simulink model "AC_Voltage_Controller"  (R2023b)
settings: Solver=VariableStepAuto  StartTime=0.0  StopTime=0.1  RelTol=1e-3
libraries: spsThyristorLib x6, spsCurrentMeasurementLib x4, spsRMSLib x4, spsVoltageMeasurementLib x4, spsSeriesRLCBranchLib x3, spsTHDLib x2, spsThreePhaseProgrammableVoltageSourceLib x1, sps_lib x1
settings Model: Creator=Anusha  LastModifiedBy=Anusha

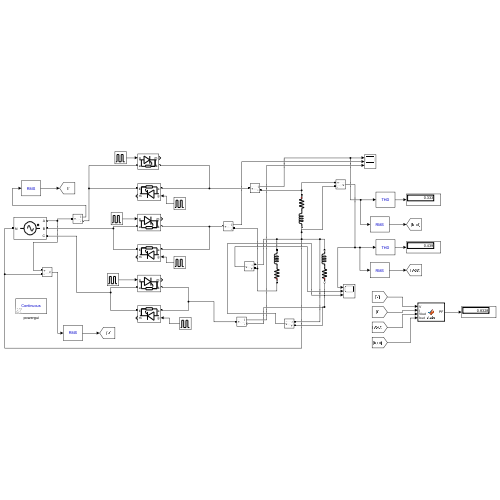
[thumbnail: Simulink's stored preview of the top-level diagram]
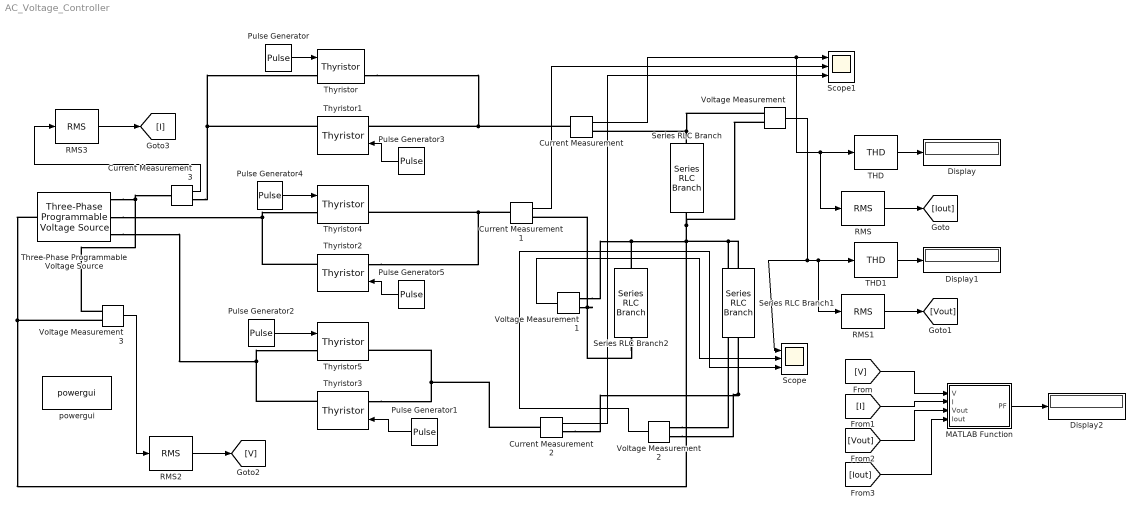
== system AC_Voltage_Controller ==
  Current Measurement{,1..3} (4 alike) : spsCurrentMeasurementLib/Current Measurement  PhasorSimulation=off  OutputType=Complex  PSBequivalent=0
  Display : Display
  Display1 : Display
  Display2 : Display
  MATLAB Function : MATLAB Function  TreatAsAtomicUnit=on
  Pulse Generator : DiscretePulseGenerator  PulseType=Time based  Period=0.02  PulseWidth=33.333  PhaseDelay=(60)*0.02/360
  Pulse Generator1 : DiscretePulseGenerator  PulseType=Time based  Period=0.02  PulseWidth=33.333  PhaseDelay=(240+180+60)*0.02/360
  Pulse Generator2 : DiscretePulseGenerator  PulseType=Time based  Period=0.02  PulseWidth=33.333  PhaseDelay=(240+60)*0.02/360
  Pulse Generator3 : DiscretePulseGenerator  PulseType=Time based  Period=0.02  PulseWidth=33.333  PhaseDelay=(180+60)*0.02/360
  Pulse Generator4 : DiscretePulseGenerator  PulseType=Time based  Period=0.02  PulseWidth=33.333  PhaseDelay=(120+60)*0.02/360
  Pulse Generator5 : DiscretePulseGenerator  PulseType=Time based  Period=0.02  PulseWidth=5  PhaseDelay=(120+180+60)*0.02/360
  RMS{,1..3} (4 alike) : spsRMSLib/RMS  TrueRMS=off  Freq=50  RMSInit=120  Ts=0
  Scope : Scope  NumInputPorts=3
  Scope1 : Scope  NumInputPorts=3
  Series RLC Branch : spsSeriesRLCBranchLib/Series RLC Branch  LConnTagsString=__new0  RConnTagsString=__new0  BranchType=RL  Resistance=1  Inductance=1e-3  SetiL0=off  InitialCurrent=0  Capacitance=1e-6  Setx0=off  InitialVoltage=0  Measurements=None
  Series RLC Branch1 : spsSeriesRLCBranchLib/Series RLC Branch  LConnTagsString=__new0  RConnTagsString=__new0  BranchType=RL  Resistance=1  Inductance=1e-3  SetiL0=off  InitialCurrent=0  Capacitance=1e-6  Setx0=off  InitialVoltage=0  Measurements=None
  Series RLC Branch2 : spsSeriesRLCBranchLib/Series RLC Branch  LConnTagsString=__new0  RConnTagsString=__new0  BranchType=RL  Resistance=1  Inductance=1e-3  SetiL0=off  InitialCurrent=0  Capacitance=1e-6  Setx0=off  InitialVoltage=0  Measurements=None
  THD : spsTHDLib/THD  Freq=60  Ts=0
  THD1 : spsTHDLib/THD  Freq=60  Ts=0
  Three-Phase Programmable Voltage Source : spsThreePhaseProgrammableVoltageSourceLib/Three-Phase Programmable Voltage Source  PositiveSequence="[311  0 50]"  VariationEntity=None  VariationType=Table of time-amplitude pairs  VariationTypeAlt=Step  VariationStep=0.5  VariationRate=10  VariationMagnitude=0.3  VariationFrequency=2  VariationTiming=[1 2]  VariationPhaseA=off  Amplitudes=[1 0.8 1.2 1.0]  TimeValues=[0 0.1 0.15 0.2]  HarmonicGeneration=off  HarmonicA=[3 0.2 -25 0]  HarmonicB=[2 0.15 35 2]  Timing="[0.05  3]"  BusType=swing  Pref=0  Qref=0  Qmin=-inf  Qmax=inf
  Thyristor{,1..5} (6 alike) : spsThyristorLib/Thyristor  Ron=0.001  Lon=0  Vf=0.8  IC=0  Rs=500  Cs=250e-9  Measurements=on
  Voltage Measurement{,1..3} (4 alike) : spsVoltageMeasurementLib/Voltage Measurement  PhasorSimulation=off  OutputType=Complex  PSBequivalent=0
  powergui : sps_lib/powergui  Priority=1  SimulationMode=Continuous  SampleTime=50e-6  frequency=60  Iterations=50  frequencyindice=50  Pbase=100e6  ErrMax=1e-4  UnitsV=kV  UnitsW=MW  buscounter=0  FunctionMessages=off  echomessages=off  EnableUseOfTLC=off  CurrentSourceSwitches=off  DisableSnubberDevices=off  DisableRonSwitches=off  DisableVfSwitches=off  DisplayEquations=off  AutomaticDiscreteSolvers=off  SolverType=Tustin/Backward Euler (TBE)  Interpol=off  ExternalGateDelay=off  methode=off  Ts=100  x0status=blocks  SPID=on  SwTol=0  HookPort=off  NonlinearTolerance=1e-4  nMaxIteration=100  ContinueOnMaxIteration=off  RestoreLinks=warning  ResistiveCurrentMeasurement=off  Frange=[0:2:500]  Ylog=off  Xlog=on  ShowGrid=off  save=off  variable=ZData  structure=0  ZoomFFT=off  StartTime=0.0  cycles=1  DisplayStyle=1  fundamental=60  FreqAxis=off  MaxFrequency=1000  frequencyindicesteady=1  RmsSteady=1  display=off
  wires:
  Pulse Generator1/1 -> Thyristor3/1
  Pulse Generator/1 -> Thyristor/1
  Pulse Generator3/1 -> Thyristor1/1
  Pulse Generator4/1 -> Thyristor4/1
  Pulse Generator5/1 -> Thyristor2/1
  Pulse Generator2/1 -> Thyristor5/1
  Voltage Measurement/1 -> RMS1/1, THD1/1, Scope/1
  Voltage Measurement1/1 -> Scope/2
  Voltage Measurement2/1 -> Scope/3
  Current Measurement1/1 -> Scope1/2
  Current Measurement2/1 -> Scope1/3
  Current Measurement/1 -> RMS/1, THD/1, Scope1/1
  THD1/1 -> Display1/1
  THD/1 -> Display/1
  Voltage Measurement3/1 -> RMS2/1
  Current Measurement3/1 -> RMS3/1
  RMS2/1 -> [V]
  RMS3/1 -> [I]
  RMS/1 -> [Iout]
  RMS1/1 -> [Vout]
  [V] -> MATLAB Function/1(V)
  [I] -> MATLAB Function/2(I)
  [Vout] -> MATLAB Function/3(Vout)
  [Iout] -> MATLAB Function/4(Iout)
  MATLAB Function/1(PF) -> Display2/1
  connections:
  Series RLC Branch2/RConn1 -- Voltage Measurement1/LConn2 -- Voltage Measurement3/LConn2 -- Three-Phase Programmable Voltage Source/LConn1 -- Series RLC Branch1/RConn1 -- Voltage Measurement2/LConn2 -- Voltage Measurement/LConn2 -- Series RLC Branch/RConn1
  Three-Phase Programmable Voltage Source/RConn1 -- Voltage Measurement3/LConn1 -- Current Measurement3/LConn1
  Thyristor2/RConn1 -- Three-Phase Programmable Voltage Source/RConn2 -- Thyristor4/LConn1
  Thyristor3/RConn1 -- Three-Phase Programmable Voltage Source/RConn3 -- Thyristor5/LConn1
  Thyristor/RConn1 -- Current Measurement/LConn1 -- Thyristor1/LConn1
  Thyristor2/LConn1 -- Current Measurement1/LConn1 -- Thyristor4/RConn1
  Thyristor3/LConn1 -- Current Measurement2/LConn1 -- Thyristor5/RConn1
  Voltage Measurement2/LConn1 -- Series RLC Branch1/LConn1 -- Current Measurement2/RConn1
  Voltage Measurement1/LConn1 -- Series RLC Branch2/LConn1 -- Current Measurement1/RConn1
  Series RLC Branch/LConn1 -- Voltage Measurement/LConn1 -- Current Measurement/RConn1
  Current Measurement3/RConn1 -- Thyristor/LConn1 -- Thyristor1/RConn1

== matlab function AC_Voltage_Controller/MATLAB Function ==
  data: V input; PF output; I input; Vout input; Iout input
function PF = stats(V,I,Vout,Iout)

Po=(Vout*Iout);
P=(V*I);
PF=(Po/P);
